simulink model "sensorModel"  (R2018b)
settings: Solver=FixedStepAuto  StartTime=0.0  StopTime=10.0  RelTol=1e-3
model workspace (MAT data in the model file):
  gpsModel = gpsSensor
  gpsModel.any.ClassNameForLoadTimeEval = 'gpsSensor'
  gpsModel.any.MajorVersionNumber = 9
  gpsModel.any.MinorVersionNumber = 1280
  gpsModel.any.ChildClassData.UpdateRate = 1
  gpsModel.any.ChildClassData.ReferenceLocation = [50.953549 -1.36553 10.5]
  gpsModel.any.ChildClassData.HorizontalPositionAccuracy = 1.6
  gpsModel.any.ChildClassData.VerticalPositionAccuracy = 3
  gpsModel.any.ChildClassData.VelocityAccuracy = 0.1
  gpsModel.any.ChildClassData.RandomStream = 'Global stream'
  gpsModel.any.ChildClassData.Seed = 7463
  gpsModel.any.ChildClassData.DecayFactor = 0.999
  gpsModel.any.SuperClassData = []
  magVar = Simulink.Parameter
  magVar.Value = -1.3
  magVar.DataType = 'auto'
  magVar.Dimensions = [1 1]
undefined symbols (not defined in the file or in its folder): Discrete, Time
libraries: ctrlSharedLib x8, simulink x4, sharedTrackingLibrary x2, aerolibnav x2, dspstat3 x1
settings Model: Creator=Aliak  LastModifiedBy=Aliak
settings DebuggingCC: ParameterUnderflowMsg=error  UniqueDataStoreMsg=warning
settings RTWCC: CheckMdlBeforeBuild=Warning

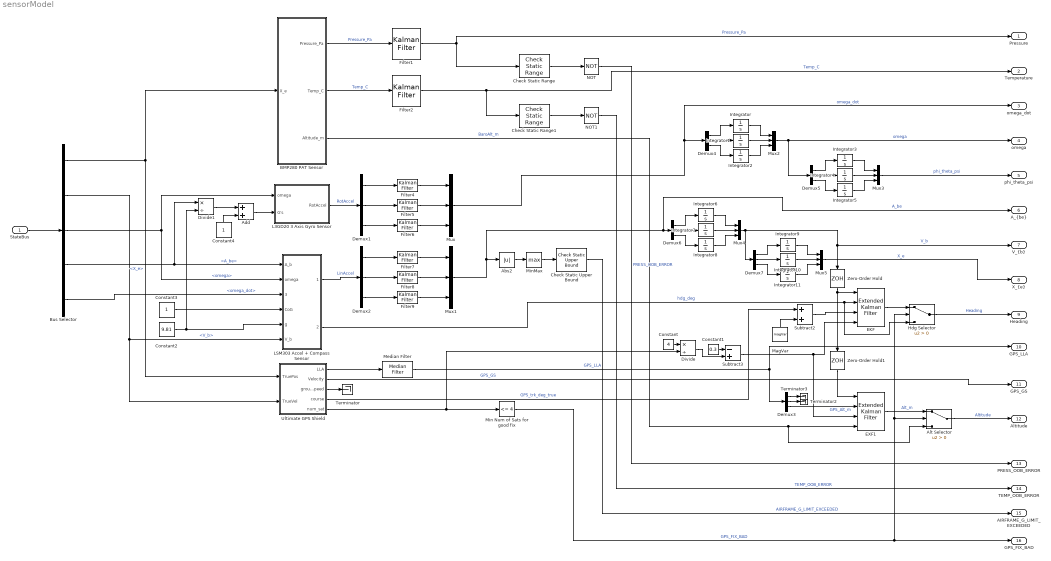
== system sensorModel ==
  StateBus : Inport  OutDataTypeStr=Bus: States
  Abs2 : Abs
  Add : Sum
  Alt Selector : Switch  Criteria=u2 > Threshold  OutDataTypeStr=single  SaturateOnIntegerOverflow=on  InputSameDT=on
  "BMP280 PAT Sensor " : Subsystem
  Bus Selector : BusSelector  OutputSignals=X_e,V_b,omega,A_be,omega_dot
  Check Static Range : simulink/Model Verification/Check  Static Range  Description=97025 <= u <= 104325  max=104325  max_included=on  min=97025  min_included=on  enabled=off  stopWhenAssertionFail=off  export=on  icon=graphic
      settings: SourceProductName=Simulink  SourceProductBaseCode=SL
  Check Static Range1 : simulink/Model Verification/Check  Static Range  Description=-10 <= u <= 30  max=30  max_included=on  min=-10  min_included=on  enabled=off  stopWhenAssertionFail=off  export=on  icon=graphic
      settings: SourceProductName=Simulink  SourceProductBaseCode=SL
  Check Static Upper Bound : simulink/Model Verification/Check Static  Upper Bound  Description=u <= 5  max=5  max_included=on  enabled=off  stopWhenAssertionFail=off  export=on  icon=graphic
      settings: SourceProductName=Simulink  SourceProductBaseCode=SL
  Constant : Constant  Value=4
  Constant1 : Constant  Value=0.3
  Constant2 : Constant  Value=9.81
  Constant3 : Constant
  Constant4 : Constant
  Demux{1..7} (7 alike) : Demux  Outputs=3
  Divide : Product  Inputs=*/  OutMin=0.5  OutMax=30  OutDataTypeStr=Inherit: Inherit via back propagation  SaturateOnIntegerOverflow=on
  Divide1 : Product  Inputs=*/
  EKF : sharedTrackingLibrary/Extended Kalman Filter  StateTransitionFcn=headingStateTransitionFunc  HasStateTransitionJacobianFcn=off  HasAdditiveProcessNoise=Additive  ProcessNoise=1  HasTimeVaryingProcessNoise=off  HasStateTransitionFcnExtraArgument=1  InitialState=0  InitialStateCovariance=3  MeasurementFcn1=baroMeasurementFunc  HasMeasurementJacobianFcn1=off  HasMeasurementEnablePort1=off  HasAdditiveMeasurementNoise1=Additive  MeasurementNoise1=0.5  HasTimeVaryingMeasurementNoise1=off  HasMeasurementFcnExtraArgument1=0  MeasurementFcn2=gpsMeasurementFunc  HasMeasurementJacobianFcn2=off  HasMeasurementEnablePort2=off  HasAdditiveMeasurementNoise2=Additive  MeasurementNoise2=1  HasTimeVaryingMeasurementNoise2=on  HasMeasurementFcnExtraArgument2=0  MeasurementFcn3=myMeasurementFcn  HasMeasurementJacobianFcn3=off  HasMeasurementEnablePort3=off  HasAdditiveMeasurementNoise3=Additive  MeasurementNoise3=1  HasTimeVaryingMeasurementNoise3=off  HasMeasurementFcnExtraArgument3=0  MeasurementFcn4=myMeasurementFcn  HasMeasurementJacobianFcn4=off  HasMeasurementEnablePort4=off  HasAdditiveMeasurementNoise4=Additive  MeasurementNoise4=1  HasTimeVaryingMeasurementNoise4=off  HasMeasurementFcnExtraArgument4=0  MeasurementFcn5=myMeasurementFcn  HasMeasurementJacobianFcn5=off  HasMeasurementEnablePort5=off  HasAdditiveMeasurementNoise5=Additive  MeasurementNoise5=1  HasTimeVaryingMeasurementNoise5=off  HasMeasurementFcnExtraArgument5=0  EnableMultirate=on  StateTransitionFcnSampleTime=0.01  MeasurementFcn1SampleTime=0.01  MeasurementFcn2SampleTime=1  MeasurementFcn3SampleTime=1  MeasurementFcn4SampleTime=1  MeasurementFcn5SampleTime=1  UseCurrentEstimator=on  OutputStateCovariance=off  DataType=double  SampleTime=1  NumberOfMeasurements=2
      settings: SourceProductName=Control System Toolbox  SourceProductBaseCode=CT
  EXF1 : sharedTrackingLibrary/Extended Kalman Filter  StateTransitionFcn=altitudeStateTransitionFunc  HasStateTransitionJacobianFcn=off  HasAdditiveProcessNoise=Additive  ProcessNoise=1  HasTimeVaryingProcessNoise=off  HasStateTransitionFcnExtraArgument=1  InitialState=0  InitialStateCovariance=1  MeasurementFcn1=gpsMeasurementFunc  HasMeasurementJacobianFcn1=off  HasMeasurementEnablePort1=off  HasAdditiveMeasurementNoise1=Additive  MeasurementNoise1=1  HasTimeVaryingMeasurementNoise1=on  HasMeasurementFcnExtraArgument1=0  MeasurementFcn2=baroMeasurementFunc  HasMeasurementJacobianFcn2=off  HasMeasurementEnablePort2=off  HasAdditiveMeasurementNoise2=Additive  MeasurementNoise2=0.8  HasTimeVaryingMeasurementNoise2=off  HasMeasurementFcnExtraArgument2=0  MeasurementFcn3=myMeasurementFcn  HasMeasurementJacobianFcn3=off  HasMeasurementEnablePort3=off  HasAdditiveMeasurementNoise3=Additive  MeasurementNoise3=1  HasTimeVaryingMeasurementNoise3=off  HasMeasurementFcnExtraArgument3=0  MeasurementFcn4=myMeasurementFcn  HasMeasurementJacobianFcn4=off  HasMeasurementEnablePort4=off  HasAdditiveMeasurementNoise4=Additive  MeasurementNoise4=1  HasTimeVaryingMeasurementNoise4=off  HasMeasurementFcnExtraArgument4=0  MeasurementFcn5=myMeasurementFcn  HasMeasurementJacobianFcn5=off  HasMeasurementEnablePort5=off  HasAdditiveMeasurementNoise5=Additive  MeasurementNoise5=1  HasTimeVaryingMeasurementNoise5=off  HasMeasurementFcnExtraArgument5=0  EnableMultirate=off  StateTransitionFcnSampleTime=0.01  MeasurementFcn1SampleTime=1  MeasurementFcn2SampleTime=1  MeasurementFcn3SampleTime=1  MeasurementFcn4SampleTime=1  MeasurementFcn5SampleTime=1  UseCurrentEstimator=on  OutputStateCovariance=off  DataType=double  SampleTime=1  NumberOfMeasurements=2
      settings: SourceProductName=Control System Toolbox  SourceProductBaseCode=CT
  Filter1 : ctrlSharedLib/Kalman Filter  TimeDomain=Discrete-Time  UseCurrentEstimator=on  ModelSource=LTI State-Space Variable  ModelSourceVariable=ss(1,[],1,[],1)  A=0.95  B=1  C=1  D=0  NumberOfStates=1  NumberOfInputs=1  NumberOfOutputs=1  InitialEstimateSource=Dialog  X0=101325  P0=10  UseK=off  UseGH=off  NumberOfProcessNoiseInputs=1  G=1  TimeInvariantG=on  H=0  TimeInvariantH=on  Q=0.05  TimeInvariantQ=on  R=1  TimeInvariantR=on  N=0  TimeInvariantN=on  AddInputPort=off  AddEnablePort=off  OutputEstimatedY=off  OutputP=off  Ts=-1
      settings: SourceProductBaseCode=CT
  Filter2 : ctrlSharedLib/Kalman Filter  TimeDomain=Discrete-Time  UseCurrentEstimator=on  ModelSource=LTI State-Space Variable  ModelSourceVariable=ss(1,[],1,[],1)  A=0.95  B=1  C=1  D=0  NumberOfStates=1  NumberOfInputs=1  NumberOfOutputs=1  InitialEstimateSource=Dialog  X0=15  P0=10  UseK=off  UseGH=off  NumberOfProcessNoiseInputs=1  G=1  TimeInvariantG=on  H=0  TimeInvariantH=on  Q=0.05  TimeInvariantQ=on  R=1  TimeInvariantR=on  N=0  TimeInvariantN=on  AddInputPort=off  AddEnablePort=off  OutputEstimatedY=off  OutputP=off  Ts=-1
      settings: SourceProductBaseCode=CT
  Filter4 : ctrlSharedLib/Kalman Filter  TimeDomain=Discrete-Time  UseCurrentEstimator=on  ModelSource=LTI State-Space Variable  ModelSourceVariable=ss(0.95,[],1,[],1/95)  A=0.95  B=1  C=1  D=0  NumberOfStates=1  NumberOfInputs=1  NumberOfOutputs=1  InitialEstimateSource=Dialog  X0=0  P0=10  UseK=off  UseGH=off  NumberOfProcessNoiseInputs=1  G=1  TimeInvariantG=on  H=0  TimeInvariantH=on  Q=0.05  TimeInvariantQ=on  R=0.8  TimeInvariantR=on  N=0  TimeInvariantN=on  AddInputPort=off  AddEnablePort=off  OutputEstimatedY=off  OutputP=off  Ts=-1
      settings: SourceProductBaseCode=CT
  Filter5 : ctrlSharedLib/Kalman Filter  TimeDomain=Discrete-Time  UseCurrentEstimator=on  ModelSource=LTI State-Space Variable  ModelSourceVariable=ss(0.95,[],1,[],1/95)  A=0.95  B=1  C=1  D=0  NumberOfStates=1  NumberOfInputs=1  NumberOfOutputs=1  InitialEstimateSource=Dialog  X0=0  P0=10  UseK=off  UseGH=off  NumberOfProcessNoiseInputs=1  G=1  TimeInvariantG=on  H=0  TimeInvariantH=on  Q=0.05  TimeInvariantQ=on  R=0.8  TimeInvariantR=on  N=0  TimeInvariantN=on  AddInputPort=off  AddEnablePort=off  OutputEstimatedY=off  OutputP=off  Ts=-1
      settings: SourceProductBaseCode=CT
  Filter6 : ctrlSharedLib/Kalman Filter  TimeDomain=Discrete-Time  UseCurrentEstimator=on  ModelSource=LTI State-Space Variable  ModelSourceVariable=ss(0.95,[],1,[],1/95)  A=0.95  B=1  C=1  D=0  NumberOfStates=1  NumberOfInputs=1  NumberOfOutputs=1  InitialEstimateSource=Dialog  X0=0  P0=10  UseK=off  UseGH=off  NumberOfProcessNoiseInputs=1  G=1  TimeInvariantG=on  H=0  TimeInvariantH=on  Q=0.05  TimeInvariantQ=on  R=0.8  TimeInvariantR=on  N=0  TimeInvariantN=on  AddInputPort=off  AddEnablePort=off  OutputEstimatedY=off  OutputP=off  Ts=-1
      settings: SourceProductBaseCode=CT
  Filter7 : ctrlSharedLib/Kalman Filter  TimeDomain=Discrete-Time  UseCurrentEstimator=on  ModelSource=LTI State-Space Variable  ModelSourceVariable=ss(0.95,[],1,[],1/100)  A=0.95  B=1  C=1  D=0  NumberOfStates=1  NumberOfInputs=1  NumberOfOutputs=1  InitialEstimateSource=Dialog  X0=0  P0=10  UseK=off  UseGH=off  NumberOfProcessNoiseInputs=1  G=1  TimeInvariantG=on  H=0  TimeInvariantH=on  Q=0.05  TimeInvariantQ=on  R=1  TimeInvariantR=on  N=0  TimeInvariantN=on  AddInputPort=off  AddEnablePort=off  OutputEstimatedY=off  OutputP=off  Ts=-1
      settings: SourceProductBaseCode=CT
  Filter8 : ctrlSharedLib/Kalman Filter  TimeDomain=Discrete-Time  UseCurrentEstimator=on  ModelSource=LTI State-Space Variable  ModelSourceVariable=ss(0.95,[],1,[],1/100)  A=0.95  B=1  C=1  D=0  NumberOfStates=1  NumberOfInputs=1  NumberOfOutputs=1  InitialEstimateSource=Dialog  X0=0  P0=10  UseK=off  UseGH=off  NumberOfProcessNoiseInputs=1  G=1  TimeInvariantG=on  H=0  TimeInvariantH=on  Q=0.05  TimeInvariantQ=on  R=1  TimeInvariantR=on  N=0  TimeInvariantN=on  AddInputPort=off  AddEnablePort=off  OutputEstimatedY=off  OutputP=off  Ts=-1
      settings: SourceProductBaseCode=CT
  Filter9 : ctrlSharedLib/Kalman Filter  TimeDomain=Discrete-Time  UseCurrentEstimator=on  ModelSource=LTI State-Space Variable  ModelSourceVariable=ss(0.95,[],1,[],1/100)  A=0.95  B=1  C=1  D=0  NumberOfStates=1  NumberOfInputs=1  NumberOfOutputs=1  InitialEstimateSource=Dialog  X0=0  P0=10  UseK=off  UseGH=off  NumberOfProcessNoiseInputs=1  G=1  TimeInvariantG=on  H=0  TimeInvariantH=on  Q=0.05  TimeInvariantQ=on  R=1  TimeInvariantR=on  N=0  TimeInvariantN=on  AddInputPort=off  AddEnablePort=off  OutputEstimatedY=off  OutputP=off  Ts=-1
      settings: SourceProductBaseCode=CT
  Hdg Selector : Switch  Criteria=u2 > Threshold  OutDataTypeStr=Inherit: Inherit via back propagation  SaturateOnIntegerOverflow=on  InputSameDT=on
  Integrator{,1..11} (12 alike) : Integrator
  L3GD20 3 Axis Gyro Sensor : Subsystem
  LSM303 Accel + Compass Sensor : Subsystem
  MagVar : Constant  Value=magVar
  Median Filter : dspstat3/Median Filter  WindowLength=20  SimulateUsing=Code generation
      settings: SourceProductName=DSP System Toolbox  SourceProductBaseCode=DS
  Min Num of Sats for good fix : simulink/Logic and Bit Operations/Compare To Constant  relop=<=  const=4  OutDataTypeStr=boolean
  MinMax : MinMax  Function=max
  Mux{,1..5} (6 alike) : Mux  Inputs=3
  NOT : Logic  Operator=NOT  IconShape=distinctive  AllPortsSameDT=off  OutDataTypeStr=boolean
  NOT1 : Logic  Operator=NOT  IconShape=distinctive  AllPortsSameDT=off  OutDataTypeStr=boolean
  Subtract2 : Sum
  Subtract3 : Sum  Inputs=-+
  Terminator : Terminator
  Terminator2 : Terminator
  Terminator3 : Terminator
  Ultimate GPS Shield : Subsystem
  Zero-Order Hold : ZeroOrderHold  SampleTime=1/100
  Zero-Order Hold1 : ZeroOrderHold
  Pressure : Outport  Unit=Pa
  Temperature : Outport  Port=2  Unit=°C
  omega_dot : Outport  Port=3  Unit=rad/s^2
  omega : Outport  Port=4  Unit=rad/s
  phi_theta_psi : Outport  Port=5  Unit=rad
  "A_{be}" : Outport  Port=6  Unit=m/s^2
  "V_{b}" : Outport  Port=7  Unit=m/s
  "X_{e}" : Outport  Port=8  Unit=m
  Heading : Outport  Port=9  Unit=deg
  GPS_LLA : Outport  Port=10
  GPS_GS : Outport  Port=11  Unit=kn
  Altitude : Outport  Port=12  Unit=m
  PRESS_OOB_ERROR : Outport  Port=13
  TEMP_OOB_ERROR : Outport  Port=14
  AIRFRAME_G_LIMIT_EXCEEDED : Outport  Port=15
  GPS_FIX_BAD : Outport  Port=16
  wires:
  Ultimate GPS Shield/4(course) -> Subtract2/1  "GPS_trk_deg_true"
  LSM303 Accel + Compass Sensor/2(hdg_deg) -> EKF/2, Hdg Selector/3  "hdg_deg"
  Ultimate GPS Shield/2(Velocity) -> GPS_GS/1  "GPS_GS"
  "BMP280 PAT Sensor "/1(Pressure_Pa) -> Filter1/1  "Pressure_Pa"
  Check Static Range/1 -> NOT/1
  NOT/1 -> PRESS_OOB_ERROR/1  "PRESS_OOB_ERROR"
  NOT1/1 -> TEMP_OOB_ERROR/1  "TEMP_OOB_ERROR"
  Check Static Range1/1 -> NOT1/1
  "BMP280 PAT Sensor "/2(Temp_C) -> Filter2/1  "Temp_C"
  Mux/1 -> omega_dot/1, Demux4/1  "omega_dot"
  "BMP280 PAT Sensor "/3(Altitude_m) -> EXF1/4, Alt Selector/3  "BaroAlt_m"
  Median Filter/1 -> GPS_LLA/1, Demux3/1  "GPS_LLA"
  Mux1/1 -> "A_{be}"/1, Demux6/1, Abs2/1  "A_be"
  Abs2/1 -> MinMax/1
  MinMax/1 -> Check Static Upper Bound/1
  Check Static Upper Bound/1 -> AIRFRAME_G_LIMIT_EXCEEDED/1  "AIRFRAME_G_LIMIT_EXCEEDED"
  Filter2/1 -> Temperature/1, Check Static Range1/1  "Temp_C"
  L3GD20 3 Axis Gyro Sensor/1(RotAccel) -> Demux1/1  "RotAccel"
  Demux1/1 -> Filter4/1
  Filter4/1 -> Mux/1
  Demux1/2 -> Filter5/1
  Filter5/1 -> Mux/2
  Demux1/3 -> Filter6/1
  Filter6/1 -> Mux/3
  Demux2/3 -> Filter9/1
  Filter9/1 -> Mux1/3
  Demux2/1 -> Filter7/1
  Filter8/1 -> Mux1/2
  Filter7/1 -> Mux1/1
  Demux2/2 -> Filter8/1
  LSM303 Accel + Compass Sensor/1(LinAccel) -> Demux2/1  "LinAccel"
  MagVar/1 -> Subtract2/2
  Subtract2/1 -> EKF/3
  Hdg Selector/1 -> Heading/1  "Heading"
  Ultimate GPS Shield/5(num_sat) -> Divide/2, Min Num of Sats for good fix/1
  Min Num of Sats for good fix/1 -> GPS_FIX_BAD/1, Hdg Selector/2, Alt Selector/2  "GPS_FIX_BAD"
  EXF1/1 -> Alt Selector/1  "Alt_m"
  Demux3/3 -> EXF1/2  "GPS_Alt_m"
  Demux3/2 -> Terminator2/1
  Demux3/1 -> Terminator3/1
  Alt Selector/1 -> Altitude/1  "Altitude"
  Ultimate GPS Shield/1(LLA) -> Median Filter/1
  EKF/1 -> Hdg Selector/1
  Demux4/1 -> Integrator/1
  Demux4/2 -> Integrator1/1
  Demux4/3 -> Integrator2/1
  Integrator/1 -> Mux2/1
  Integrator1/1 -> Mux2/2
  Integrator2/1 -> Mux2/3
  Mux2/1 -> Demux5/1, omega/1  "omega"
  Demux5/1 -> Integrator3/1
  Demux5/2 -> Integrator4/1
  Integrator3/1 -> Mux3/1
  Demux5/3 -> Integrator5/1
  Integrator4/1 -> Mux3/2
  Integrator5/1 -> Mux3/3
  Mux3/1 -> phi_theta_psi/1  "phi_theta_psi"
  Integrator7/1 -> Mux4/2
  Integrator11/1 -> Mux5/3
  Integrator10/1 -> Mux5/2
  Demux7/2 -> Integrator10/1
  Integrator9/1 -> Mux5/1
  Mux5/1 -> "X_{e}"/1  "X_e"
  Demux6/1 -> Integrator6/1
  Demux6/3 -> Integrator8/1
  Demux7/3 -> Integrator11/1
  Integrator8/1 -> Mux4/3
  Mux4/1 -> Demux7/1, "V_{b}"/1, Zero-Order Hold/1  "V_b"
  Demux6/2 -> Integrator7/1
  Demux7/1 -> Integrator9/1
  Integrator6/1 -> Mux4/1
  Constant/1 -> Divide/1
  Divide/1 -> Subtract3/2
  Constant1/1 -> Subtract3/1
  Subtract3/1 -> EXF1/3, EKF/4
  Zero-Order Hold/1 -> Zero-Order Hold1/1, EKF/1
  Zero-Order Hold1/1 -> EXF1/1
  Filter1/1 -> Pressure/1, Check Static Range/1  "Pressure_Pa"
  Constant2/1 -> LSM303 Accel + Compass Sensor/5(g), Divide1/2
  StateBus/1 -> Bus Selector/1
  Constant3/1 -> LSM303 Accel + Compass Sensor/4(CoG)
  Bus Selector/1 -> Ultimate GPS Shield/1(TruePos), "BMP280 PAT Sensor "/1(X_e)  "<X_e>"
  Bus Selector/2 -> Ultimate GPS Shield/2(TrueVel), LSM303 Accel + Compass Sensor/6(V_b)  "<V_b>"
  Bus Selector/3 -> L3GD20 3 Axis Gyro Sensor/1(omega), LSM303 Accel + Compass Sensor/2(omega)  "<omega>"
  Bus Selector/5 -> LSM303 Accel + Compass Sensor/3(omega_dot)  "<omega_dot>"
  Bus Selector/4 -> Divide1/1, LSM303 Accel + Compass Sensor/1(A_b)  "<A_be>"
  Divide1/1 -> Add/1
  Add/1 -> L3GD20 3 Axis Gyro Sensor/2(G's)
  Constant4/1 -> Add/2
  Ultimate GPS Shield/3(groundspeed) -> Terminator/1

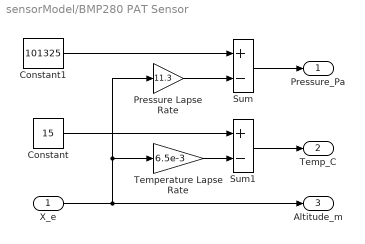
== system sensorModel/BMP280 PAT Sensor  ==
  X_e : Inport  Unit=m
  Constant : Constant  Value=15
  Constant1 : Constant  Value=101325
  Pressure Lapse Rate : Gain  Gain=11.3
  Sum : Sum  Inputs=+-
  Sum1 : Sum  Inputs=+-
  Temperature Lapse Rate : Gain  Gain=6.5e-3
  Pressure_Pa : Outport  Unit=Pa
  Temp_C : Outport  Port=2  Unit=°C
  Altitude_m : Outport  Port=3  Unit=m
  wires:
  Constant1/1 -> Sum/1
  Sum/1 -> Pressure_Pa/1
  X_e/1 -> Altitude_m/1, Pressure Lapse Rate/1, Temperature Lapse Rate/1
  Pressure Lapse Rate/1 -> Sum/2
  Sum1/1 -> Temp_C/1
  Constant/1 -> Sum1/1
  Temperature Lapse Rate/1 -> Sum1/2

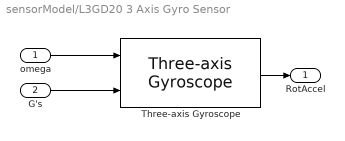
== system sensorModel/L3GD20 3 Axis Gyro Sensor ==
  omega : Inport
  G's : Inport  Port=2
  Three-axis Gyroscope : aerolibnav/Three-axis Gyroscope  dtype_g=on  w_g=190  z_g=0.707  g_sf_cc=[1 0 0; 0 1 0; 0 0 1]  g_bias=[0 0 0]  g_sen=[0 0 0]  g_Ts=0  g_rand=on  g_seeds=[23093 23094 23095]  g_pow=[0.0001 0.0001 0.0001]  g_sat="[-inf  -inf  -inf  inf inf inf]"
      settings: SourceProductName=Aerospace Blockset  SourceProductBaseCode=AE
  RotAccel : Outport  Unit=rad/s^2
  wires:
  Three-axis Gyroscope/1 -> RotAccel/1
  omega/1 -> Three-axis Gyroscope/1
  G's/1 -> Three-axis Gyroscope/2

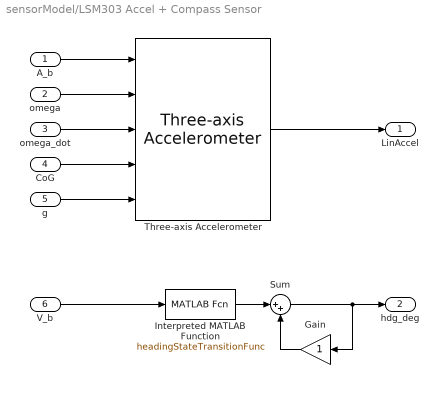
== system sensorModel/LSM303 Accel + Compass Sensor ==
  A_b : Inport
  omega : Inport  Port=2
  omega_dot : Inport  Port=3
  CoG : Inport  Port=4
  g : Inport  Port=5
  V_b : Inport  Port=6
  Gain : Gain
  Interpreted MATLAB Function : MATLABFcn  MATLABFcn=headingStateTransitionFunc  OutputDimensions=1
  Sum : Sum  Inputs=|++
  Three-axis Accelerometer : aerolibnav/Three-axis Accelerometer  units=Metric (MKS)  acc=[0 0 0]  gtype=on  dtype_a=on  w_a=190  z_a=0.707  a_sf_cc=[1 0 0; 0 1 0; 0 0 1]  a_bias=[0 0 0]  a_Ts=0  a_rand=on  a_seeds=[23093 23094 23095]  a_pow=[0.001 0.001 0.001]  a_sat="[-inf  -inf  -inf  inf inf inf]"
      settings: SourceProductName=Aerospace Blockset  SourceProductBaseCode=AE
  LinAccel : Outport  Unit=m/s^2
  hdg_deg : Outport  Port=2  Unit=deg
  wires:
  Three-axis Accelerometer/1 -> LinAccel/1
  V_b/1 -> Interpreted MATLAB Function/1
  A_b/1 -> Three-axis Accelerometer/1
  omega/1 -> Three-axis Accelerometer/2
  CoG/1 -> Three-axis Accelerometer/4
  g/1 -> Three-axis Accelerometer/5
  Interpreted MATLAB Function/1 -> Sum/1
  Sum/1 -> Gain/1, hdg_deg/1
  Gain/1 -> Sum/2
  omega_dot/1 -> Three-axis Accelerometer/3

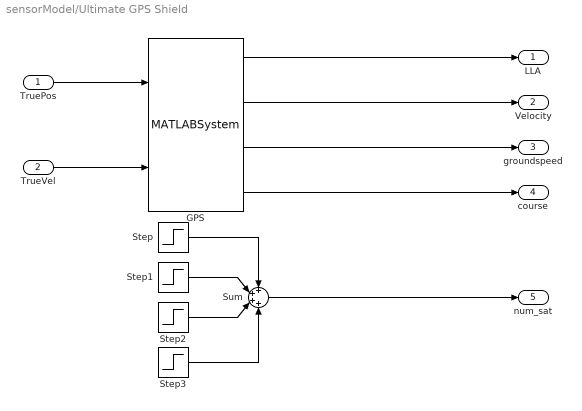
== system sensorModel/Ultimate GPS Shield ==
  TruePos : Inport  PortDimensions=3
  TrueVel : Inport  Port=2  PortDimensions=3
  GPS : MATLABSystem  System=gpsSensor  UpdateRate=1  ReferenceLocation=[50.953549 -1.365530 10.5]  HorizontalPositionAccuracy=1.6  VerticalPositionAccuracy=3  VelocityAccuracy=0.1  RandomStream=Global stream  Seed=uint32( 67 )  DecayFactor=0.999  SimulateUsing=Code generation
      mask Type: gpsSensor
      mask Display:
      | disp('gpsSensor');
      | port_label('input',1,'pos');
      | port_label('input',2,'vel');
      | port_label('output',1,'llaMeas');
      | port_label('output',2,'velMeas');
      | port_label('output',3,'groundspeedMeas');
      | port_label('output',4,'courseMeas');
  Step : Step  Time=10  SampleTime=0
  Step1 : Step  Time=15  SampleTime=0
  Step2 : Step  Time=25  SampleTime=0
  Step3 : Step  Time=40  SampleTime=0
  Sum : Sum  Inputs=++++
  LLA : Outport
  Velocity : Outport  Port=2  Unit=m/s
  groundspeed : Outport  Port=3  Unit=kn
  course : Outport  Port=4  Unit=deg
  num_sat : Outport  Port=5
  wires:
  GPS/1 -> LLA/1
  GPS/2 -> Velocity/1
  GPS/4 -> course/1
  Sum/1 -> num_sat/1
  GPS/3 -> groundspeed/1
  Step/1 -> Sum/1
  Step1/1 -> Sum/2
  Step2/1 -> Sum/3
  Step3/1 -> Sum/4
  TruePos/1 -> GPS/1
  TrueVel/1 -> GPS/2
